simulink model "sampleModel1889_3_sub_sub"  (R2023a)
settings: Solver=VariableStepAuto  StartTime=0.0  StopTime=10.0  RelTol=1e-3
libraries: hdlsllib x8, simulink x4
settings Model: Creator=user1  LastModifiedBy=user1

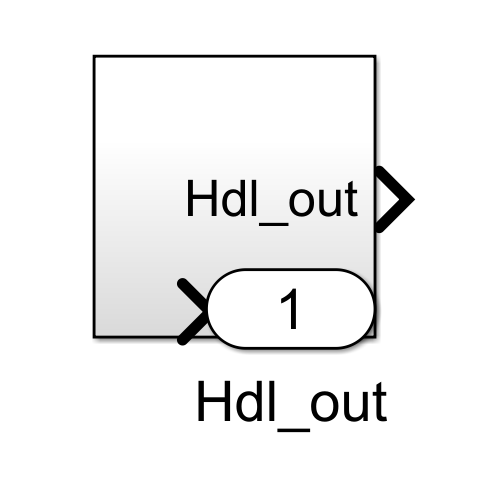
[thumbnail: Simulink's stored preview of the top-level diagram]
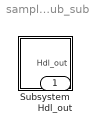
== system sampleModel1889_3_sub_sub ==
  Subsystem : Subsystem
  Hdl_out : Outport  OutDataTypeStr=uint8

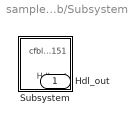
== system sampleModel1889_3_sub_sub/Subsystem ==
  Subsystem : Subsystem
  Hdl_out : Outport  OutDataTypeStr=uint8

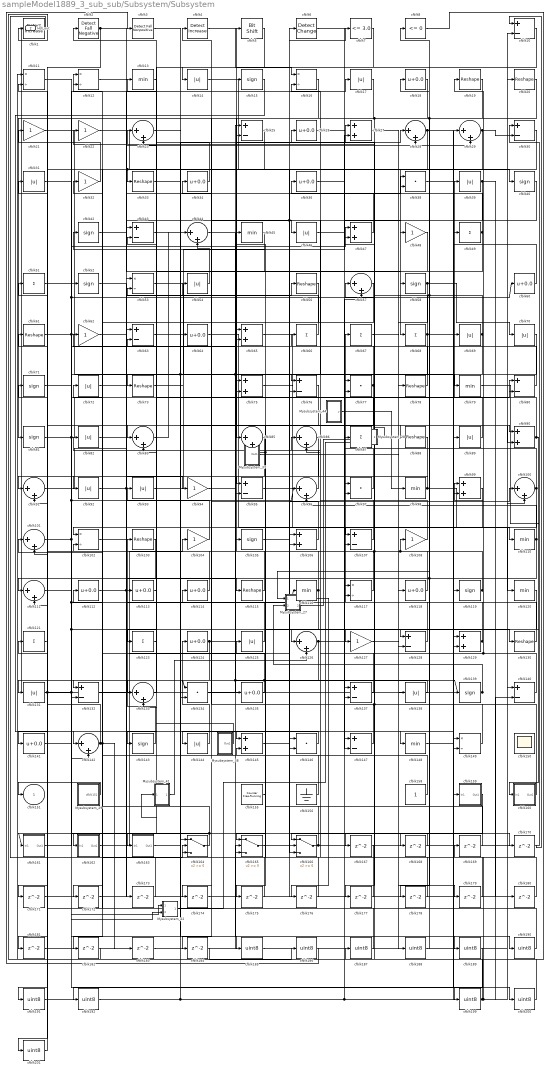
== system sampleModel1889_3_sub_sub/Subsystem/Subsystem ==
  Mysubsystem_22 : Subsystem  TreatAsAtomicUnit=on  RTWFcnName=Mysubsystem_22
      settings: RTWFcnNameOpts=User specified  RTWFileNameOpts=Use function name
  Mysubsystem_27 : Subsystem  TreatAsAtomicUnit=on  RTWFcnName=Mysubsystem_27
      settings: RTWFcnNameOpts=User specified  RTWFileNameOpts=Use function name
  Mysubsystem_28 : Subsystem  TreatAsAtomicUnit=on  RTWFcnName=Mysubsystem_28
      settings: RTWFcnNameOpts=User specified  RTWFileNameOpts=Use function name
  Mysubsystem_29 : Subsystem  TreatAsAtomicUnit=on  RTWFcnName=Mysubsystem_29
      settings: RTWFcnNameOpts=User specified  RTWFileNameOpts=Use function name
  Mysubsystem_37 : Subsystem  TreatAsAtomicUnit=on  RTWFcnName=Mysubsystem_37
      settings: RTWFcnNameOpts=User specified  RTWFileNameOpts=Use function name
  Mysubsystem_38 : Subsystem  TreatAsAtomicUnit=on  RTWFcnName=Mysubsystem_38
      settings: RTWFcnNameOpts=User specified  RTWFileNameOpts=Use function name
  Mysubsystem_41 : Subsystem  TreatAsAtomicUnit=on  RTWFcnName=Mysubsystem_41
      settings: RTWFcnNameOpts=User specified  RTWFileNameOpts=Use function name
  Mysubsystem_44 : Subsystem  TreatAsAtomicUnit=on  RTWFcnName=Mysubsystem_44
      settings: RTWFcnNameOpts=User specified  RTWFileNameOpts=Use function name
  cfblk1 : simulink/Logic and Bit Operations/Detect Increase  vinit=0.0  OutDataTypeStr=uint8
      settings: LibrarySourceBlock=|
      | hdlsllib/Logic and Bit
      | Operations/Detect
      | Increase
  cfblk{10,25,30,43,63,76,80,95,107,128,132,137,140,147} (14 alike) : Sum  Inputs=+-  OutDataTypeStr=uint8
  cfblk{23,28..29,44,57,83,85..86,91,96,100..101,111,126,133,142} (16 alike) : Sum  Inputs=|++  OutDataTypeStr=uint8
  cfblk{11..12,16,53,102,117,149} (7 alike) : Product  Inputs=*/  OutDataTypeStr=uint8  RndMeth=Zero  SaturateOnIntegerOverflow=on
  cfblk{19..20,33,56,61,73,78,88,103,115,130} (11 alike) : Reshape
  cfblk{21..22,32,48,62,94,104,108,127} (9 alike) : Gain  OutDataTypeStr=uint8
  cfblk{15,40,42,52,58,71,81,105,119,139,143} (11 alike) : Signum
  cfblk{27,47,65,75,90,99,106,129,145} (9 alike) : Sum  OutDataTypeStr=uint8
  cfblk{13,45,79,98,110,116,120,148} (8 alike) : MinMax  OutDataTypeStr=uint8
  cfblk{18,26,34,36,60,64,112..114,118,124,135,141} (13 alike) : Bias  Bias=0.0  SaturateOnIntegerOverflow=off
  cfblk{49,51,66..68,87,121,123} (8 alike) : Sum  Inputs=+  OutDataTypeStr=uint8
  cfblk{14,17,31,39,46,54,69..70,72,82,89,92..93,125,131,138,144} (17 alike) : Abs  OutDataTypeStr=uint8  SaturateOnIntegerOverflow=off
  cfblk{38,77,97,134,146} (5 alike) : DotProduct  OutDataTypeStr=uint8
  cfblk150 : Scope
      settings: Floating=on
  cfblk155 : hdlsllib/Sources/Counter Free-Running  NumBits=16  tsamp=-1
  cfblk156 : Ground
  cfblk158 : Constant  OutDataTypeStr=uint8  SampleTime=-1
  cfblk159 : Subsystem
      settings: LibrarySourceBlock=|
      | hdlsllib/Ports &
      | Subsystems/Subsystem
  cfblk160 : Subsystem
      settings: LibrarySourceBlock=|
      | hdlsllib/Ports &
      | Subsystems/Subsystem
  cfblk161 : Subsystem
      settings: LibrarySourceBlock=|
      | hdlsllib/Ports &
      | Subsystems/Subsystem
  cfblk162 : Subsystem
      settings: LibrarySourceBlock=|
      | hdlsllib/Ports &
      | Subsystems/Subsystem
  cfblk163 : Subsystem
      settings: LibrarySourceBlock=|
      | hdlsllib/Ports &
      | Subsystems/Subsystem
  cfblk164 : Switch  OutDataTypeStr=uint8  SaturateOnIntegerOverflow=off  InputSameDT=off
  cfblk165 : Switch  OutDataTypeStr=uint8  SaturateOnIntegerOverflow=off  InputSameDT=off
  cfblk166 : Switch  OutDataTypeStr=uint8  SaturateOnIntegerOverflow=off  InputSameDT=off
  cfblk{167..184} (18 alike) : Delay  SampleTime=1
  cfblk{185..192,199..201} (11 alike) : DataTypeConversion  OutDataTypeStr=uint8  SaturateOnIntegerOverflow=off  RndMeth=Floor
  cfblk2 : hdlsllib/Logic and Bit Operations/Detect Fall Negative  vinit=0  OutDataTypeStr=uint8
  cfblk3 : hdlsllib/Logic and Bit Operations/Detect Fall Nonpositive  vinit=0  OutDataTypeStr=uint8
  cfblk4 : simulink/Logic and Bit Operations/Detect Increase  vinit=0.0  OutDataTypeStr=uint8
      settings: LibrarySourceBlock=|
      | hdlsllib/Logic and Bit
      | Operations/Detect
      | Increase
  cfblk5 : hdlsllib/Logic and Bit Operations/Bit Shift  mode=Shift Left Logical  N=0
  cfblk6 : simulink/Logic and Bit Operations/Detect Change  vinit=0  OutDataTypeStr=uint8
      settings: LibrarySourceBlock=|
      | hdlsllib/Logic and Bit
      | Operations/Detect
      | Change
  cfblk7 : hdlsllib/Logic and Bit Operations/Compare To Constant  relop=<=  const=3.0  OutDataTypeStr=uint8
  cfblk8 : hdlsllib/Logic and Bit Operations/Compare To Zero  relop=<=  OutDataTypeStr=uint8
  cfblk151 : Outport  OutDataTypeStr=uint8  VectorParamsAs1DForOutWhenUnconnected=off
  Hdl_out : Outport  Port=2  OutDataTypeStr=uint8
  wires:
  Mysubsystem_44/1(y) -> cfblk98/1
  Mysubsystem_41/1(Out1) -> cfblk126/2
  Mysubsystem_38/1(Out1) -> Mysubsystem_41/1(In1)
  Mysubsystem_37/1(Out1) -> cfblk118/1
  Mysubsystem_29/1(cfblk151) -> cfblk151/1
  Mysubsystem_28/1(Out1) -> cfblk177/1
  Mysubsystem_22/1(Out1) -> Mysubsystem_28/2(In2)
  Mysubsystem_27/2(Out2) -> Mysubsystem_28/1(In1)
  Mysubsystem_27/1(Out1) -> cfblk176/1
  cfblk139/1 -> Mysubsystem_27/2(In2), Hdl_out/1
  cfblk201/1 -> cfblk11/2
  cfblk200/1 -> cfblk11/1
  cfblk199/1 -> cfblk169/1, cfblk140/2, cfblk107/2
  cfblk192/1 -> cfblk20/1
  cfblk189/1 -> cfblk192/1
  cfblk191/1 -> cfblk149/1, cfblk97/1, cfblk64/1
  cfblk190/1 -> cfblk51/1
  cfblk51/1 -> cfblk189/1
  cfblk188/1 -> cfblk8/1
  cfblk127/1 -> cfblk188/1
  cfblk187/1 -> cfblk112/1
  cfblk8/1 -> cfblk187/1
  cfblk186/1 -> cfblk3/1
  cfblk184/1 -> cfblk186/1
  cfblk185/1 -> cfblk69/1
  cfblk3/1 -> cfblk185/1
  cfblk18/1 -> cfblk184/1
  cfblk183/1 -> cfblk100/2
  cfblk182/1 -> cfblk1/1
  cfblk181/1 -> cfblk165/2
  cfblk180/1 -> cfblk86/2
  cfblk179/1 -> cfblk147/1
  cfblk67/1 -> cfblk179/1
  cfblk178/1 -> cfblk145/2
  cfblk177/1 -> cfblk53/1
  cfblk176/1 -> cfblk102/2
  cfblk175/1 -> cfblk164/1
  cfblk76/1 -> cfblk175/1
  cfblk174/1 -> cfblk106/1
  cfblk173/1 -> cfblk63/1
  cfblk62/1 -> cfblk173/1
  cfblk172/1 -> cfblk140/1
  cfblk57/1 -> cfblk172/1
  cfblk171/1 -> cfblk43/1
  cfblk170/1 -> cfblk10/1
  cfblk23/1 -> cfblk170/1
  cfblk169/1 -> cfblk146/1
  cfblk168/1 -> cfblk166/1
  cfblk159/1(Out1) -> cfblk168/1
  cfblk167/1 -> cfblk164/3
  cfblk125/1 -> cfblk54/1
  cfblk39/1 -> cfblk76/1, cfblk180/1
  cfblk112/1 -> cfblk56/1, cfblk167/1
  cfblk53/1 -> cfblk166/2
  cfblk49/1 -> cfblk133/2, cfblk16/2
  cfblk96/1 -> cfblk42/1
  cfblk12/1 -> cfblk46/1
  cfblk66/1 -> cfblk23/2
  cfblk92/1 -> cfblk148/1, cfblk38/2
  cfblk115/1 -> cfblk13/1
  cfblk94/1 -> cfblk38/1
  cfblk60/1 -> cfblk49/1
  cfblk99/1 -> cfblk132/1
  cfblk133/1 -> cfblk93/1
  cfblk149/1 -> cfblk114/1
  cfblk147/1 -> cfblk86/1
  cfblk156/1 -> cfblk125/1
  cfblk85/1 -> cfblk101/2
  cfblk131/1 -> Mysubsystem_22/2(In2), cfblk80/2, cfblk96/1, cfblk116/1, cfblk61/1
  cfblk108/1 -> cfblk77/1
  cfblk137/1 -> cfblk23/1
  cfblk145/1 -> cfblk100/1
  cfblk104/1 -> cfblk83/2
  cfblk63/1 -> cfblk89/1
  cfblk36/1 -> cfblk48/1
  cfblk120/1 -> cfblk137/2
  cfblk121/1 -> cfblk141/1
  cfblk87/1 -> cfblk26/1
  cfblk111/1 -> cfblk142/2
  cfblk88/1 -> cfblk95/1
  cfblk31/1 -> cfblk128/1
  cfblk95/1 -> cfblk159/1(In1)
  cfblk45/1 -> cfblk65/2
  cfblk119/1 -> cfblk108/1, cfblk12/1, cfblk99/1
  cfblk107/1 -> cfblk62/1
  cfblk70/1 -> cfblk117/2
  cfblk165/1 -> cfblk28/2
  cfblk77/1 -> cfblk111/2, cfblk12/2
  cfblk27/1 -> cfblk40/1
  cfblk30/1 -> cfblk106/2
  cfblk26/1 -> cfblk137/1
  cfblk155/1 -> cfblk85/2, cfblk45/1
  cfblk138/1 -> cfblk133/1
  cfblk61/1 -> cfblk63/2, cfblk166/3
  cfblk113/1 -> cfblk163/1(In1)
  cfblk52/1 -> cfblk94/1
  cfblk68/1 -> cfblk132/2, cfblk165/3, cfblk22/1, cfblk200/1
  cfblk56/1 -> cfblk146/2
  cfblk19/1 -> cfblk134/2, cfblk107/1, cfblk178/1
  cfblk161/1(Out1) -> cfblk60/1, cfblk15/1
  cfblk38/1 -> cfblk129/1
  cfblk6/1 -> cfblk79/1
  cfblk65/1 -> cfblk90/2
  cfblk166/1 -> cfblk30/1, cfblk75/1
  cfblk101/1 -> cfblk52/1, cfblk149/2
  cfblk102/1 -> cfblk115/1
  cfblk86/1 -> cfblk92/1
  cfblk135/1 -> cfblk32/1, cfblk134/1
  cfblk73/1 -> cfblk27/2
  cfblk116/1 -> cfblk105/1, cfblk165/1
  cfblk93/1 -> cfblk25/1
  cfblk128/1 -> cfblk113/1
  cfblk134/1 -> cfblk80/1, cfblk139/1
  cfblk4/1 -> cfblk16/1
  cfblk100/1 -> cfblk147/2, cfblk57/1
  cfblk22/1 -> cfblk78/1
  cfblk91/1 -> cfblk17/1
  cfblk69/1 -> cfblk18/1, cfblk25/2, cfblk95/2
  cfblk72/1 -> cfblk127/1
  cfblk75/1 -> cfblk119/1
  cfblk46/1 -> cfblk117/1
  cfblk44/1 -> cfblk135/1
  cfblk21/1 -> cfblk138/1
  cfblk163/1(Out1) -> cfblk28/1
  cfblk71/1 -> cfblk65/1
  cfblk80/1 -> cfblk47/2
  cfblk42/1 -> cfblk29/2
  cfblk43/1 -> cfblk145/1, cfblk75/2
  cfblk132/1 -> cfblk6/1
  cfblk110/1 -> Mysubsystem_27/1(In1), cfblk162/1(In1), cfblk96/2
  cfblk123/1 -> cfblk53/2
  cfblk20/1 -> cfblk191/1
  cfblk82/1 -> cfblk130/1
  cfblk34/1 -> cfblk2/1
  cfblk28/1 -> cfblk90/1, cfblk181/1
  cfblk29/1 -> cfblk102/1, cfblk30/2
  cfblk58/1 -> cfblk70/1, cfblk128/2
  cfblk25/1 -> cfblk33/1, cfblk201/1
  cfblk140/1 -> cfblk82/1, cfblk99/2
  cfblk129/1 -> cfblk19/1, cfblk97/2
  cfblk32/1 -> cfblk21/1
  cfblk11/1 -> cfblk199/1
  cfblk103/1 -> cfblk111/1
  cfblk105/1 -> cfblk7/1
  cfblk5/1 -> cfblk14/1
  cfblk40/1 -> cfblk76/2, cfblk174/1
  cfblk130/1 -> cfblk87/1
  cfblk148/1 -> cfblk29/1
  cfblk14/1 -> cfblk68/1
  cfblk89/1 -> cfblk43/2
  cfblk48/1 -> cfblk73/1
  cfblk47/1 -> cfblk36/1
  cfblk2/1 -> cfblk91/2, cfblk58/1
  cfblk160/1(Out1) -> cfblk27/1, cfblk66/1
  cfblk54/1 -> cfblk44/2
  cfblk16/1 -> cfblk85/1
  cfblk90/1 -> cfblk39/1, cfblk160/1(In1)
  cfblk118/1 -> cfblk31/1, cfblk77/2
  cfblk124/1 -> cfblk131/1, cfblk190/1
  cfblk33/1 -> cfblk88/1
  cfblk81/1 -> Mysubsystem_22/1(In1), cfblk129/2, cfblk10/2
  cfblk13/1 -> cfblk123/1
  cfblk141/1 -> cfblk47/1
  cfblk144/1 -> cfblk124/1
  cfblk117/1 -> cfblk5/1
  cfblk158/1 -> cfblk101/1
  cfblk143/1 -> cfblk103/1
  cfblk97/1 -> cfblk67/1
  cfblk10/1 -> cfblk83/1
  cfblk78/1 -> cfblk4/1
  cfblk114/1 -> cfblk71/1
  cfblk7/1 -> cfblk143/1
  cfblk1/1 -> cfblk164/2
  cfblk142/1 -> cfblk182/1, cfblk183/1, cfblk121/1
  cfblk164/1 -> cfblk72/1, cfblk161/1(In1)
  cfblk106/1 -> cfblk34/1
  cfblk146/1 -> cfblk144/1
  cfblk98/1 -> cfblk91/1, cfblk120/1
  cfblk126/1 -> cfblk57/2, cfblk171/1
  cfblk15/1 -> cfblk142/1
  cfblk83/1 -> cfblk44/1
  cfblk79/1 -> cfblk126/1
  cfblk17/1 -> cfblk81/1
  cfblk64/1 -> cfblk110/1
  cfblk162/1(Out1) -> cfblk104/1

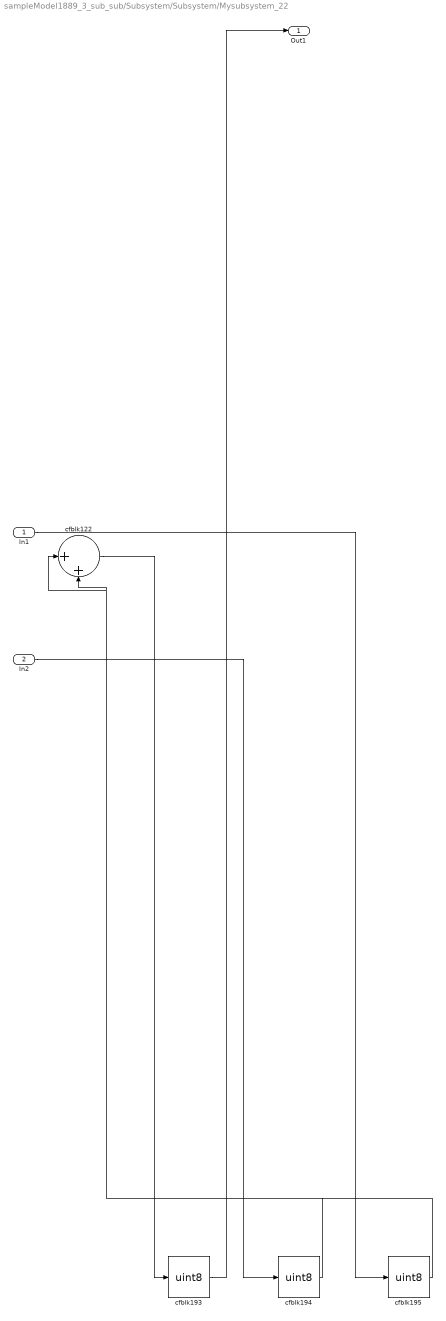
== system sampleModel1889_3_sub_sub/Subsystem/Subsystem/Mysubsystem_22 ==
  In1 : Inport
  In2 : Inport  Port=2
  cfblk122 : Sum  Inputs=|++
  cfblk193 : DataTypeConversion  OutDataTypeStr=uint8  SaturateOnIntegerOverflow=off  RndMeth=Floor
  cfblk194 : DataTypeConversion  OutDataTypeStr=uint8  SaturateOnIntegerOverflow=off  RndMeth=Floor
  cfblk195 : DataTypeConversion  OutDataTypeStr=uint8  SaturateOnIntegerOverflow=off  RndMeth=Floor
  Out1 : Outport
  wires:
  cfblk122/1 -> cfblk193/1
  cfblk194/1 -> cfblk122/1
  cfblk195/1 -> cfblk122/2
  cfblk193/1 -> Out1/1
  In2/1 -> cfblk194/1
  In1/1 -> cfblk195/1

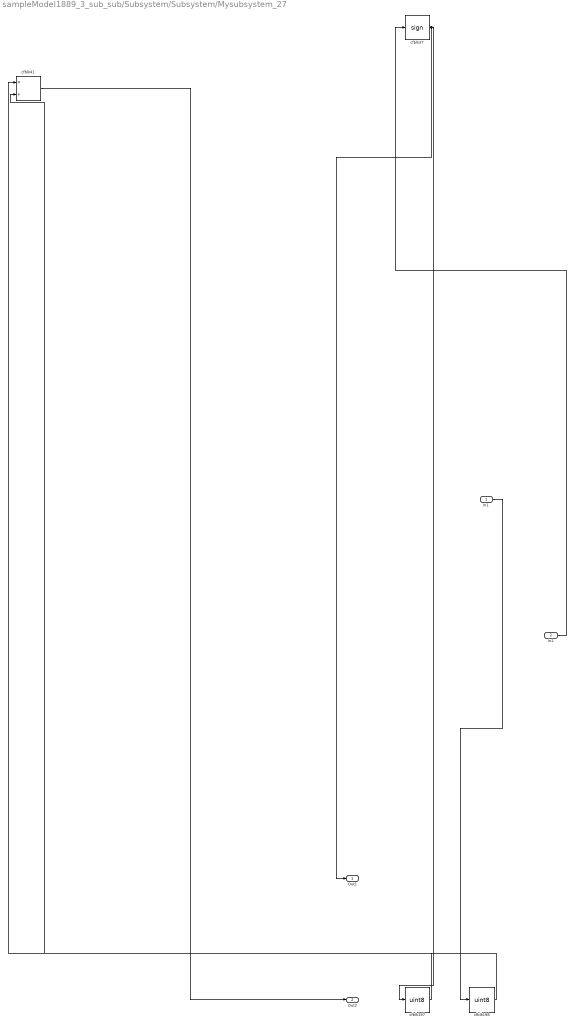
== system sampleModel1889_3_sub_sub/Subsystem/Subsystem/Mysubsystem_27 ==
  In1 : Inport
  In2 : Inport  Port=2
  cfblk197 : DataTypeConversion  OutDataTypeStr=uint8  SaturateOnIntegerOverflow=off  RndMeth=Floor
  cfblk198 : DataTypeConversion  OutDataTypeStr=uint8  SaturateOnIntegerOverflow=off  RndMeth=Floor
  cfblk37 : Signum
  cfblk41 : Product  Inputs=*/  RndMeth=Zero  SaturateOnIntegerOverflow=on
  Out1 : Outport
  Out2 : Outport  Port=2
  wires:
  In2/1 -> cfblk37/1
  cfblk197/1 -> cfblk41/1
  cfblk37/1 -> Out1/1, cfblk197/1
  In1/1 -> cfblk198/1
  cfblk198/1 -> cfblk41/2
  cfblk41/1 -> Out2/1

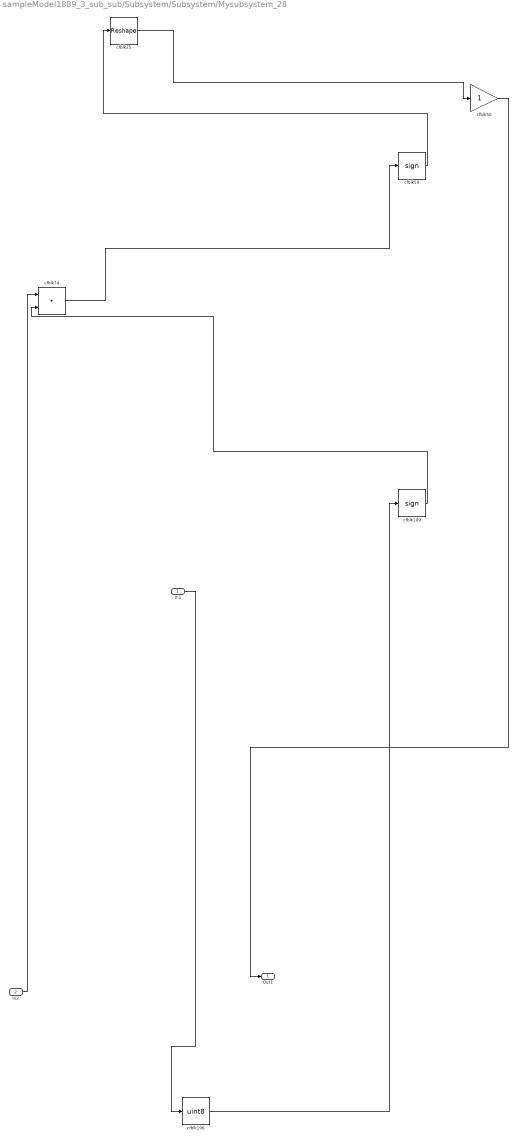
== system sampleModel1889_3_sub_sub/Subsystem/Subsystem/Mysubsystem_28 ==
  In1 : Inport
  In2 : Inport  Port=2
  cfblk109 : Signum
  cfblk196 : DataTypeConversion  OutDataTypeStr=uint8  SaturateOnIntegerOverflow=off  RndMeth=Floor
  cfblk35 : Reshape
  cfblk50 : Gain
  cfblk59 : Signum
  cfblk74 : DotProduct  OutDataTypeStr=Inherit: Inherit via internal rule
  Out1 : Outport
  wires:
  cfblk196/1 -> cfblk109/1
  cfblk109/1 -> cfblk74/2
  cfblk59/1 -> cfblk35/1
  In1/1 -> cfblk196/1
  In2/1 -> cfblk74/1
  cfblk74/1 -> cfblk59/1
  cfblk50/1 -> Out1/1
  cfblk35/1 -> cfblk50/1

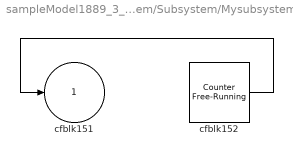
== system sampleModel1889_3_sub_sub/Subsystem/Subsystem/Mysubsystem_29 ==
  cfblk152 : hdlsllib/Sources/Counter Free-Running  NumBits=16  tsamp=-1
  cfblk151 : Outport  VectorParamsAs1DForOutWhenUnconnected=off
  wires:
  cfblk152/1 -> cfblk151/1

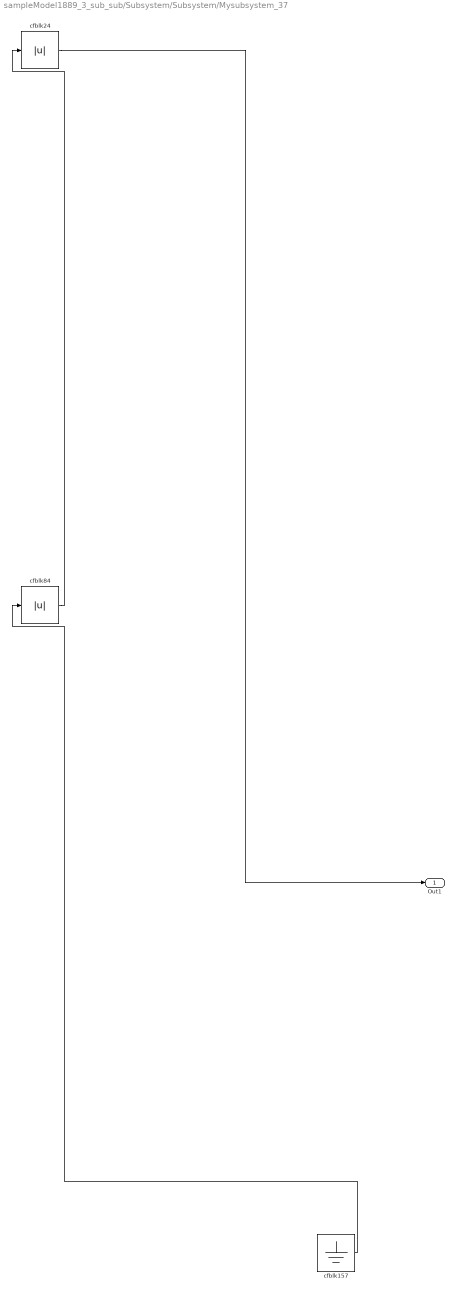
== system sampleModel1889_3_sub_sub/Subsystem/Subsystem/Mysubsystem_37 ==
  cfblk157 : Ground
  cfblk24 : Abs  SaturateOnIntegerOverflow=off
  cfblk84 : Abs  SaturateOnIntegerOverflow=off
  Out1 : Outport
  wires:
  cfblk157/1 -> cfblk84/1
  cfblk84/1 -> cfblk24/1
  cfblk24/1 -> Out1/1

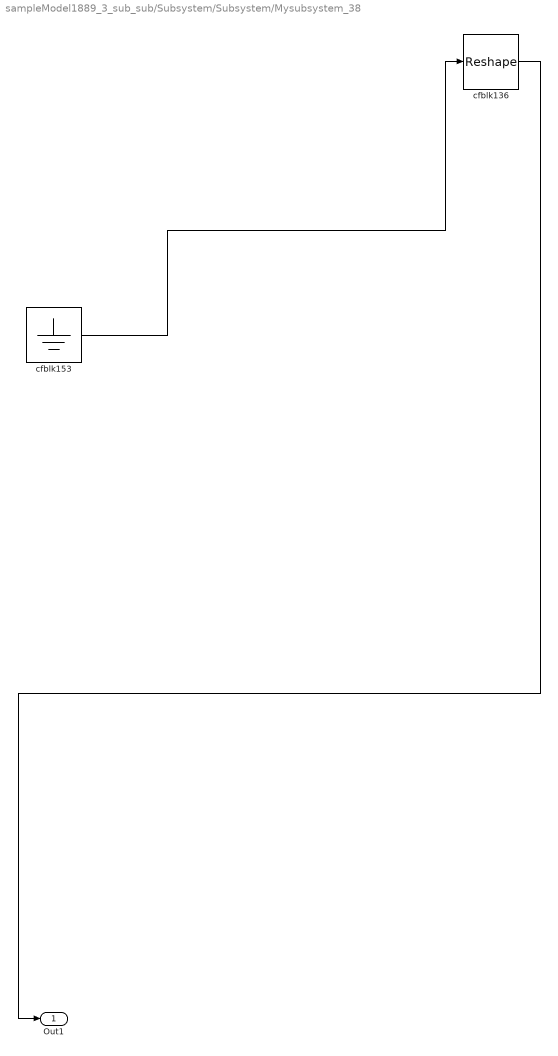
== system sampleModel1889_3_sub_sub/Subsystem/Subsystem/Mysubsystem_38 ==
  cfblk136 : Reshape
  cfblk153 : Ground
  Out1 : Outport
  wires:
  cfblk153/1 -> cfblk136/1
  cfblk136/1 -> Out1/1

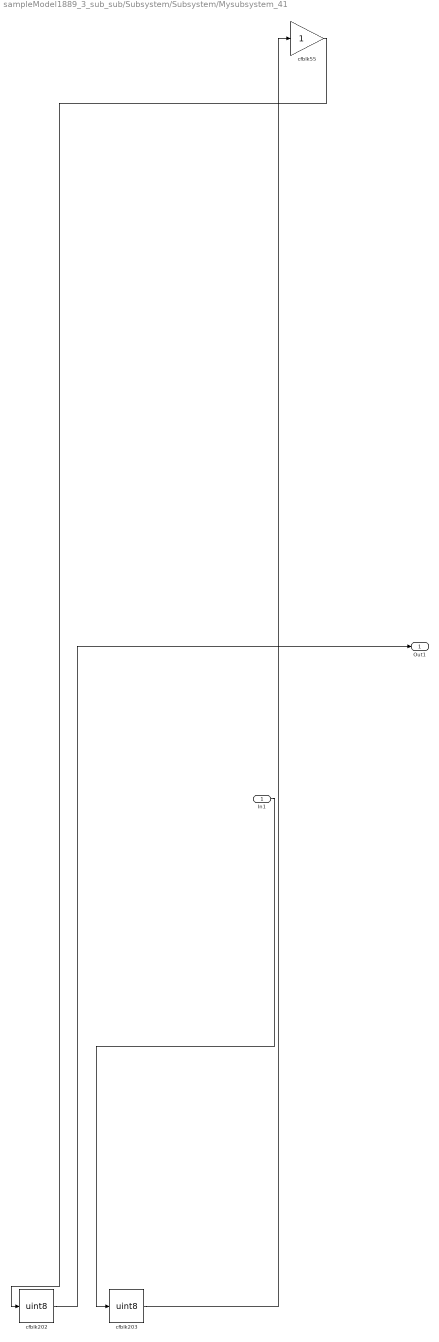
== system sampleModel1889_3_sub_sub/Subsystem/Subsystem/Mysubsystem_41 ==
  In1 : Inport
  cfblk202 : DataTypeConversion  OutDataTypeStr=uint8  SaturateOnIntegerOverflow=off  RndMeth=Floor
  cfblk203 : DataTypeConversion  OutDataTypeStr=uint8  SaturateOnIntegerOverflow=off  RndMeth=Floor
  cfblk55 : Gain
  Out1 : Outport
  wires:
  cfblk203/1 -> cfblk55/1
  cfblk55/1 -> cfblk202/1
  cfblk202/1 -> Out1/1
  In1/1 -> cfblk203/1

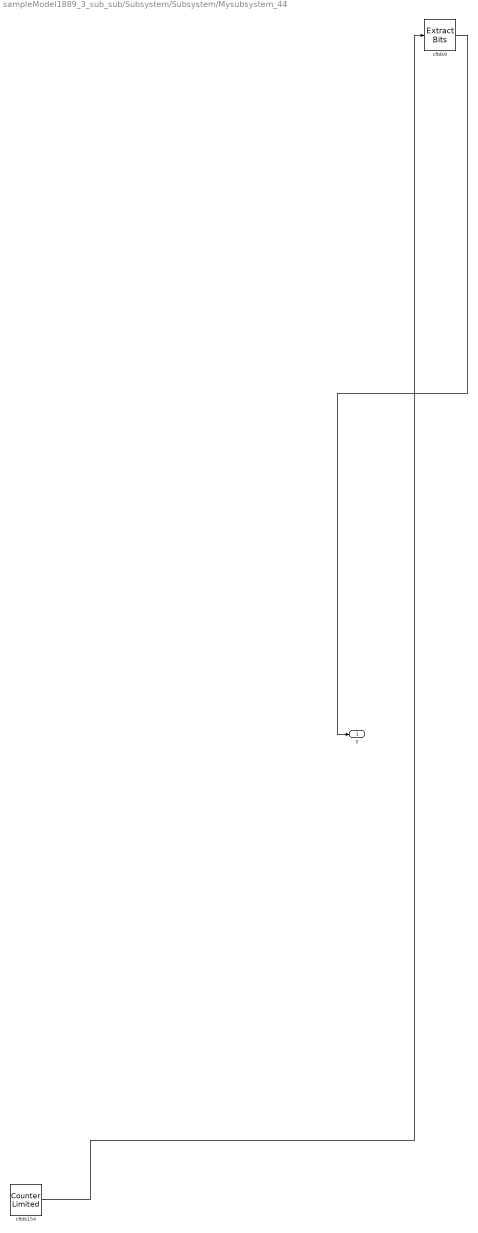
== system sampleModel1889_3_sub_sub/Subsystem/Subsystem/Mysubsystem_44 ==
  cfblk154 : hdlsllib/Sources/Counter Limited  uplimit=7  tsamp=-1
  cfblk9 : simulink/Logic and Bit Operations/Extract Bits  bitsToExtract=Upper half  numBits=8  bitIdxRange=[0 7]  outScalingMode=Preserve fixed-point scaling
      settings: LibrarySourceBlock=|
      | hdlsllib/Logic and Bit
      | Operations/Extract Bits
  y : Outport
  wires:
  cfblk154/1 -> cfblk9/1
  cfblk9/1 -> y/1

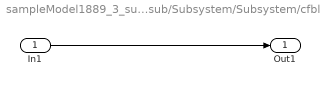
== system sampleModel1889_3_sub_sub/Subsystem/Subsystem/cfblk159 ==
  In1 : Inport
  Out1 : Outport
  wires:
  In1/1 -> Out1/1

== system sampleModel1889_3_sub_sub/Subsystem/Subsystem/cfblk160 ==
  In1 : Inport
  Out1 : Outport
  wires:
  In1/1 -> Out1/1

== system sampleModel1889_3_sub_sub/Subsystem/Subsystem/cfblk161 ==
  In1 : Inport
  Out1 : Outport
  wires:
  In1/1 -> Out1/1

== system sampleModel1889_3_sub_sub/Subsystem/Subsystem/cfblk162 ==
  In1 : Inport
  Out1 : Outport
  wires:
  In1/1 -> Out1/1

== system sampleModel1889_3_sub_sub/Subsystem/Subsystem/cfblk163 ==
  In1 : Inport
  Out1 : Outport
  wires:
  In1/1 -> Out1/1
